simulink model "staubli_20210216_18a"  (R2020a)
settings: Solver=VariableStepAuto  StartTime=0.0  StopTime=10  RelTol=1e-3
values from neighbouring files (symbols this model uses):
  s = T06(1:3,2)    [jacobian_test.m]
undefined symbols (not defined in the file or in its folder): X, Y, Z
libraries: sm_lib x37, nesl_utility x7, dsppolyfun x6, simulink x6
(part 2 of 2)

== matlab function staubli_20210216_18a/MATLAB Function ==
  data: q1 input; y output; q2 input; q3 input; q4 input; q5 input; q6 input
function y = fcn(q1,q2,q3,q4,q5,q6)

y=[q1,q2,q3,q4,q5,q6];
% % y= [q1,q2,q3,q4,q5,q6]
% d1=0.1;
% d2=0.1;
% d3=0.1;
% d4=0.1;
% d5=0.1;
% d6=0.1;
% % 
% % 
% % q1=0;
% % q2=0;
% % q3=pi/2;
% % q4=0;
% % q5=0;
% % q6=0;
% 
% q0 = 0; %% base 부터 joint1 까지 거리 
% e0 = 0; %% endeffector wrist 부터 flange 까지 거리
% tcpx = 0; %% flange 부터 tcp 까지 거리
% tcpz = 0; %% flange 부터 tcp 까지 거리
% R = 0; %% TCP 각도 0
% 
% dq1=0;
% dq2=0;
% dq3=0;
% dq4=0;
% dq5=0;
% dq6=0;
% 
% 
% 
% % l1=0.0595-0.01;%doesnt matter
% l2=0.05;
% l3=0.0506;
% l4=0.0493;
% l5=0.0507;
% l6=0.05;
% 
% m1=1.4058;
% m2=1.2209;
% m3=0.9742;
% m4=0.7446;
% m5=0.7446;
% m6=0.3853;
% 
% zz1=0.000406218509370527;
% 
% xx2=0.000311258660573173;
% yy2=0.00113057980116099;
% zz2=0.00113500164711486;
% 
% xx3=0.000195610120509242;
% yy3=0.000890675212348444;
% zz3=0.000892205392556534;
% 
% xx4=0.000661301749537305;
% yy4=0.000114515268992527;
% zz4=0.000662306036923719;
% 
% xx5=0.000661293830235689;
% yy5=0.000114514748053103;
% zz5=0.000662295948156026;
% 
% xx6=0.000336151788940896; 
% yy6=0.000336151788940896;
% zz6=3.01034757383826E-05;
% 
% % syms q0 e0 tcpx tcpz R
% % syms q1 q2 q3 q4 q5 q6
% % syms d1 d2 d3 d4 d5 d6
% g = 9.8;
% 
% T1=[cos(q1)  0  sin(q1) 0;
%     sin(q1)  0 -cos(q1) 0;
%     0        1       0  d1;
%     0        0       0   1];
% 
% T2=[cos(q2) -sin(q2) 0 d2*cos(q2);
%     sin(q2)  cos(q2) 0 d2*sin(q2);
%     0              0 1          0;
%     0              0 0          1];
% 
% T3=[cos(q3) 0 sin(q3)  d3*cos(q3);
%     sin(q3) 0 -cos(q3) d3*sin(q3);
%     0       1  0          0;
%     0       0  0          1];
% 
% T4=[cos(q4) 0 -sin(q4)  0;
%     sin(q4) 0 cos(q4)   0;
%     0       1   0       d4;
%     0       0   0       1];
% 
% T5=[cos(q5) 0 -sin(q5)  d5*cos(q5);
%     sin(q5) 0 cos(q5)   d5*sin(q5);
%     0       1  0        0;
%     0       0   0       1];
% 
% T6=[cos(q6) -sin(q6) 0  0;
%     sin(q6)  cos(q6) 0  0;
%     0           0    1  d6;
%     0           0    0  1];
% 
% Tb = [1 0 0  0;
%     0  1 0  0;
%     0  0 1  q0;
%     0  0 0  1];
% 
% Tee = [1 0 0  0;
%     0  1 0  0;
%     0  0 1  e0;
%     0  0 0  1];
% 
% Ttcp = [cos(R) 0 sin(R)  tcpx;
%     0  1 0  0;
%     -sin(R)  0 cos(R)  tcpz;
%     0  0 0  1];
%    
% T01=T1;
% T02=T1*T2;
% T03=T1*T2*T3;
% T04=T1*T2*T3*T4;
% T05=T1*T2*T3*T4*T5;
% T06=T1*T2*T3*T4*T5*T6;
% Ttcp=Tb*T06*Tee*Ttcp;
% 
% R1=[cos(q1) -sin(q1) 0; %% the i th link rotation matrix
%     sin(q1)  cos(q1) 0;
%     0           0    1];
% 
% R2=[T02(1,1:3);
%     T02(2,1:3);
%     T02(3,1:3)];
% 
% R3=[T03(1,1:3);
%     T03(2,1:3);
%     T03(3,1:3)];
% 
% R4=[T04(1,1:3);
%     T04(2,1:3);
%     T04(3,1:3)];
% 
% R5=[T05(1,1:3);
%     T05(2,1:3);
%     T05(3,1:3)];
% 
% R6=[T06(1,1:3);
%     T06(2,1:3);
%     T06(3,1:3)];
% 
% jv1=jacobian([T01(1,4),T01(2,4),T01(3,4)],[q1,q2,q3,q4,q5,q6]);
% jv2=jacobian([T02(1,4),T02(2,4),T02(3,4)],[q1,q2,q3,q4,q5,q6]);
% jv3=jacobian([T03(1,4),T03(2,4),T03(3,4)],[q1,q2,q3,q4,q5,q6]);
% jv4=jacobian([T04(1,4),T04(2,4),T04(3,4)],[q1,q2,q3,q4,q5,q6]);
% jv5=jacobian([T05(1,4),T05(2,4),T05(3,4)],[q1,q2,q3,q4,q5,q6]);
% jv6=jacobian([T06(1,4),T06(2,4),T06(3,4)],[q1,q2,q3,q4,q5,q6]);
% % 
% % syms l1 l2 l3 l4 l5 l6
% 
% JV1=[0 0 0 0 0 0;  %% upper part of jacobian matrix
%      0 0 0 0 0 0;
%      0 0 0 0 0 0];
%   
% JV2=[-l2*cos(q2)*sin(q1), -l2*cos(q1)*sin(q2),0,0,0,0;
%       l2*cos(q1)*cos(q2), -l2*sin(q1)*sin(q2),0,0,0,0;
%                        0,          l2*cos(q2),0,0,0,0];
% 
% JV3=subs(jv3,d3,l3);
% JV4=subs(jv4,d4,l4);
% JV5=subs(jv5,d5,l5);
% JV6=subs(jv6,d6,l6);
% 
% jw=[0,T1(1,3),T02(1,3),T03(1,3),T04(1,3),T05(1,3);  %% lower part of jacobian
%     0,T1(2,3),T02(2,3),T03(2,3),T04(2,3),T05(2,3);
%     1,T1(3,3),T02(3,3),T03(3,3),T04(3,3),T05(3,3)];
% 
% JW1=jw;
% JW1(:,2:6)=0;
% 
% JW2=jw;
% JW2(:,3:6)=0;
% 
% JW3=jw;
% JW3(:,4:6)=0;
% 
% JW4=jw;
% JW4(:,5:6)=0;
% 
% JW5=jw;
% JW5(:,6)=0;
% 
% JW6=jw;
% 
% % syms m1 m2 m3 m4 m5 m6
% % syms xx1 yy1 zz1 xx2 yy2 zz2 xx3 yy3 zz3
% % syms xx4 yy4 zz4 xx5 yy5 zz5 xx6 yy6 zz6
% 
% IXX=[xx1 xx2 xx3 xx4 xx5 xx6];
% IYY=[yy1 yy2 yy3 yy4 yy5 yy6];
% IZZ=[zz1 zz2 zz3 zz4 zz5 zz6];
% 
% I1=[IXX(1) 0 0; 0 IYY(1) 0; 0 0 IZZ(1)]; %% inertia tensor
% I2=[IXX(2) 0 0; 0 IYY(2) 0; 0 0 IZZ(2)];
% I3=[IXX(3) 0 0; 0 IYY(3) 0; 0 0 IZZ(3)];
% I4=[IXX(4) 0 0; 0 IYY(4) 0; 0 0 IZZ(4)];
% I5=[IXX(5) 0 0; 0 IYY(5) 0; 0 0 IZZ(5)];
% I6=[IXX(6) 0 0; 0 IYY(6) 0; 0 0 IZZ(6)];
% 
% D1=m1*JV1.'*JV1+JW1.'*R1*I1*R1.'*JW1; %% joint-space inertia matrix
% D2=m2*JV2.'*JV2+JW2.'*R2*I2*R2.'*JW2;
% D3=m3*JV3.'*JV3+JW3.'*R3*I3*R3.'*JW3;
% D4=m4*JV4.'*JV4+JW4.'*R4*I4*R4.'*JW4;
% D5=m5*JV5.'*JV5+JW5.'*R5*I5*R5.'*JW5;
% D6=m6*JV6.'*JV6+JW6.'*R6*I6*R6.'*JW6;
% 
% 
% D=D1+D2+D3+D4+D5+D6;
% % 
% % syms dq1 dq2 dq3 dq4 dq5 dq6
% 
% Q=[q1 q2 q3 q4 q5 q6]
% DQ=[dq1 dq2 dq3 dq4 dq5 dq6]
% C=sym(zeros(6)); %% Christoffel matrix, which presents the centrifugal and Coriolis terms
% for k=1:6
%     for j=1:6
%         for i=1:6
%             C(k,j)=C(k,j)+(1/2*(diff(D(k,j),Q(i))+jacobian(D(k,i),Q(j))-jacobian(D(i,j),Q(k))))*DQ(i);
%         end
%         
%     end
% end
% 
% %  % seeking gravity matrix
% %  P1 =[x1;y1;z1]; % the coordinates of centroid 1 at {1}
% %  P01 = T01([1 2 3],[1 2 3])*P1; % centroid 1 is under {0}
% % 
% %  P2 = [x2; y2; z2]; % centroid 2 at {2} coordinates
% %  P02 = T02([1 2 3],[1 2 3])*P2; % centroid 2 coordinates in {0}
% % 
% %  P3 = [x3; y3; z3]; % centroid 3 at {3} coordinates
% %  P03 = T03([1 2 3], [1 2 3])*P3; % centroid 3 coordinates in {0}
% % 
% %  P4 = [x4; y4; z4]; %coordinates of  centroid 4 at {4}
% % P04 = T04([1 2 3],[1 2 3])*P4; % centroid 4 is under {0}
% % 
% %  P5 = [x5; y5; z5]; % centroid 5 at {5} coordinates
% %  P05 = T05([1 2 3],[1 2 3])*P5; % centroid 5 is under {0}
% % 
% %  P6 = [x1; y1; z1]; %the coordinates of % centroid 6 at {6}
% %  P06 = T06([1 2 3],[1 2 3])*P6; % centroid 6 is under {0}
% % 
% %  % potential expression
% % P = m1*g*P01(3,1)+m2*g*P02(3,1)+m3*g*P03(3,1)+m4*g*P04(3,1)+m5*g*P05(3,1)+m6*g*P06(3,1);
% % 
% %  % potential can be used to guide theta1
% % G01 = diff( P,q1);
% %  % potential can be used to guide theta2
% % G02 = diff( P,q2);
% %  % potential can be used to guide theta3
% % G03 = diff( P,q3);
% %  % potential can be used to guide theta4
% % G04 = diff( P,q4);
% %  % potential can be partial to theta5
% % G05 = diff( P,q5);
% %  % potential can be used to guide theta6
% % G06 = diff( P,q6);
% % 
% %  % gravity matrix
% % G = [G01; G02; G03; G04; G05; G06];
% 
% 
% M=subs(D)
% JV=subs(jv6)
% 
% K=eye(6)*100
% range=1000;
% for tmp=1:1:range 
%     
%     w=tmp*2*pi;
%     
%     G=M*(-w^2)+K;
%   
%     FRF=JV*inv(G)*JV.';
%     
%     hxx=abs(FRF(1,1));
%     hxy=abs(FRF(2,1));
%     hxz=abs(FRF(3,1));
%     
%     hyy=abs(FRF(2,2));
%     hyz=abs(FRF(3,2));
%     
%     hzz=abs(FRF(3,3));
%     
%     
% end
% 
% 
%     plot(1:range,hxx(1:range))
%     grid on
%     legend('model','FEM') 
%     set(gca, 'YScale', 'log')
%     textobj = findobj('type', 'axes');
%             set(textobj, 'fontname', 'Times New Roman');
%             set(textobj, 'fontunits', 'points');
%             set(textobj, 'fontsize', 16);
%             set(textobj,'fontweight','bold');
%             xlim([0 500]);
% 
%     title('h_{ffxx}')
%     xlabel('frequency (Hz)')
%     ylabel('magnitude (m/N)')
% 
%     figure
%     plot(1:range,hxy(1:range))
%     grid on
%     legend('model','FEM')
%     set(gca, 'YScale', 'log')
%     textobj = findobj('type', 'axes');
%             set(textobj, 'fontname', 'Times New Roman');
%             set(textobj, 'fontunits', 'points');
%             set(textobj, 'fontsize', 16);
%             set(textobj,'fontweight','bold');
%             xlim([0 1000]);
% 
%     title('h_{ffxy}')
%     xlabel('frequency (Hz)')
%     ylabel('magnitude (m/N)')
%     
%     figure
%     plot(1:range,hxz(1:range))
%     grid on
%     legend('model','FEM')
%     set(gca, 'YScale', 'log')
%     textobj = findobj('type', 'axes');
%             set(textobj, 'fontname', 'Times New Roman');
%             set(textobj, 'fontunits', 'points');
%             set(textobj, 'fontsize', 16);
%             set(textobj,'fontweight','bold');
%             xlim([0 1000]);
% 
%     title('h_{ffxz}')
%     xlabel('frequency (Hz)')
%     ylabel('magnitude (m/N)')
% 
%     figure
%     plot(1:range,hyy(1:range))
%     grid on
%     legend('model','FEM')
%     set(gca, 'YScale', 'log')
%     textobj = findobj('type', 'axes');
%             set(textobj, 'fontname', 'Times New Roman');
%             set(textobj, 'fontunits', 'points');
%             set(textobj, 'fontsize', 16);
%             set(textobj,'fontweight','bold');
%             xlim([0 1000]);
% 
%     title('h_{ffyy}')
%     xlabel('frequency (Hz)')
%     ylabel('magnitude (m/N)')
%     
%     figure
%     plot(1:range,hyz(1:range))
%     grid on
%     legend('model','FEM')
%     set(gca, 'YScale', 'log')
%     textobj = findobj('type', 'axes');
%             set(textobj, 'fontname', 'Times New Roman');
%             set(textobj, 'fontunits', 'points');
%             set(textobj, 'fontsize', 16);
%             set(textobj,'fontweight','bold');
%             xlim([0 1000]);
% 
%     title('h_{ffyz}')
%     xlabel('frequency (Hz)')
%     ylabel('magnitude (m/N)')
% 
%     figure
%     plot(1:range,hzz(1:range))
%     grid on
%     legend('model','FEM')
%     set(gca, 'YScale', 'log')
%     textobj = findobj('type', 'axes');
%             set(textobj, 'fontname', 'Times New Roman');
%             set(textobj, 'fontunits', 'points');
%             set(textobj, 'fontsize', 16);
%             set(textobj,'fontweight','bold');
%             xlim([0 1000]);
% 
%     title('h_{ffzz}')
%     xlabel('frequency (Hz)')
%     ylabel('magnitude (m/N)')
% 
% 
% y = q1;
